simulink model "PID_Validation_Luca"  (R2024b)
settings: Solver=ode45  StartTime=0.0  StopTime=4  RelTol=1e-3
values from neighbouring files (symbols this model uses):
  Beq = mot.B+(mld.Bh)/((gbox.N)^2)    [LQR_code.m]
  Jb = 1.4e-3    (= 0.0014)    [Elastic_parameters_estimation.m]
  Kd = Kp * TD    [PID.m]
  Ki = Kp / TI    [PID.m]
  Kp = 1/(magP * magC)    [PID.m]
  Kw = 1/T_w    (= 7.14285714286)    [PID_Luca.m]
  N = linsolve(SYS,f)    [LQR_code.m]
  Req = sens.curr.Rs+mot.R    [LQR_code.m]
  tl = 1/(10*wgc)    [PID_Luca.m]
undefined symbols (not defined in the file or in its folder): Bb, daq, deg2V, drv, Jeq_hat, k, k_drv, Ke, Kt, mot, rads2rpm, sens, T_drv, tau_sf, V2deg
settings Model: Creator=Banaan  LastModifiedBy=lucag

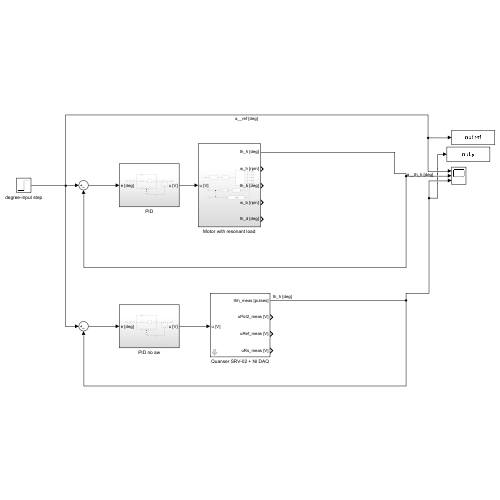
[thumbnail: Simulink's stored preview of the top-level diagram]
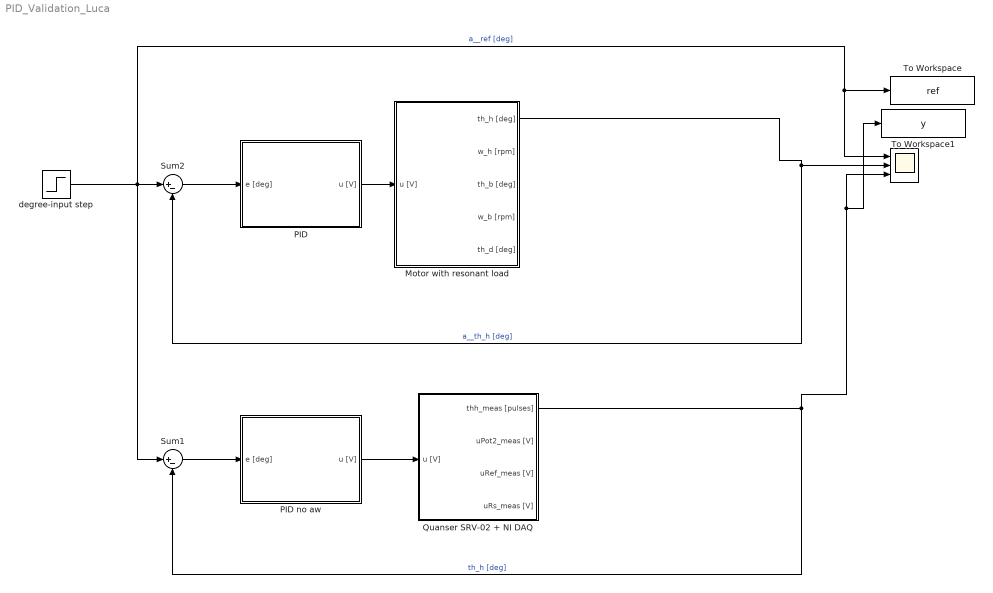
== system PID_Validation_Luca ==
  " " : Scope  NumInputPorts=3
  Motor with resonant load : Subsystem
  PID : Subsystem
  PID no aw : Subsystem
  Quanser SRV-02 + NI DAQ : Subsystem  mask(Quanser SRV-02 (with resonant load) + NI DAQ){Ts=0.001, fricType=Coulomb + viscous, lockShaft=off, beamInitPos=10}
      mask prompts: Ts "NI DAQ Sample Time:"; fricType "Friction model"; lockShaft "Lock motor shaft"; beamInitPos "Beam initial position [deg]:"
      mask help: Quanser SRV-02 (with resonant load) + NI DAQ model.
      mask init:
      | %%
      | % Riccardo Antonello (riccardo.antonello@unipd.it)
      | %
      | % April 28, 2020
      | %
      | % Dept. of Information Engineering, University of Padova
      | %
      | 
      | %%  Conversion gains
      | deg2rad = pi/180;                   %   [deg]   -> [rad]
      | rad2deg = 180/pi;                   %   [rad]   -> [deg]
      | 
      | 
      | %%  Sensors data
      | 
      | %   shunt resistor
      | sens.curr.Rs = 0.5;   
      | 
      | %   Hewlett-Packard HEDS-5540#A06 optical encoder
      | sens.enc.ppr = 500*4;                                                   %   pulses per rotation
      | sens.enc.pulse2deg = 360/sens.enc.ppr;                                  %   [pulses] -> [deg]
      | sens.enc.pulse2rad = 2*pi/sens.enc.ppr;                                 %   [pulses] -> [rad]
      | sens.enc.deg2pulse = sens.enc.ppr/360;                                  %   [deg] -> [pulses]
      | sens.enc.rad2pulse = sens.enc.ppr/2/pi;                                 %   [rad] -> [pulses]
      | 
      | %   potentiometer 2 (Spectrol 357-0-0-103) - installed on hub
      | sens.pot2.range.R      = 10e3;                                          %   ohmic value range 
      | sens.pot2.range.V      = 5;                                             %   voltage range
      | sens.pot2.range.th_deg = 340;                                           %   angle range [deg]
      | sens.pot2.range.th     = sens.pot2.range.th_deg * deg2rad;              %   angle range [rad]                           
      | sens.pot2.deg2V        = sens.pot2.range.V / sens.pot2.range.th_deg;    %   sensitivity [V/deg]
      | sens.pot2.rad2V        = sens.pot2.range.V / sens.pot2.range.th;        %   sensitivity [V/rad]
      | sens.pot2.V2deg        = 1/sens.pot2.deg2V;                             %   conversion gain [V] -> [deg]
      | sens.pot2.V2rad        = 1/sens.pot2.rad2V;                             %   conversion gain [V] -> [rad]
      | sens.pot2.noise.var    = 3.5e-7;                                        %   out noise variance [V^2]
      | 
      | 
      | %%  Data acquisition board (daq) data
      | 
      | %   NI PCI-6221 DAC data
      | daq.dac.bits = 16;                                  %   resolution (bits)
      | daq.dac.fs   = 10;                                  %   full scale 
      | daq.dac.q    = 2*daq.dac.fs/(2^daq.dac.bits-1);     %	quantization
      | 
      | %   NI PCI-6221 ADC data
      | daq.adc.bits = 16;                                  %   resolution (bits)
      | daq.adc.fs   = 10;                                  %   full scale (as set in SLDRT Analog Input block)
      | daq.adc.q    = 2*daq.adc.fs/(2^daq.adc.bits-1);     %   quantization   
      | 
      | 
      | %%  Set beam initial position
      | % SRV02Handle = find_system(gcb, ...
      | %     'LookUnderMasks', 'on', ...
      | %     'FindAll', 'on', ...
      | %     'FollowLinks', 'on', ...
      | %     'SearchDepth', '1', ...
      | %     'BlockType', 'ModelReference', ...
      | %     'Name', 'Quanser SRV-02');
      | %
      | % %get_param(SRV02Handle, 'InstanceParameters')
      | % InstanceParams = get_param(SRV02Handle, 'InstanceParameters');
      | % for k = 1:length(InstanceParams)
      | %     if strcmp(InstanceParams(k).Name, 'thb0')
      | %         if lockShaft
      | %             InstanceParams(k).Value = sprintf('%f', beamInitPos);
      | %         else
      | %             InstanceParams(k).Value = sprintf('%f', 0);    
      | %         end
      | %         set_param(SRV02Handle, 'InstanceParameters', InstanceParams);
      | %         break;
      | %     end
      | % end
      | 
      | if lockShaft
      |     thb0 = beamInitPos;
      | else
      |     thb0 = 0;    
      | end
      | 
      | 
      | %%  Mask initialization
      | if lockShaft
      |     
      |     %   find Inport handle
      |     InPortHandle = find_system(gcb, ...
      |         'LookUnderMasks', 'on', ...
      |         'FindAll', 'on', ...
      |         'FollowLinks', 'on', ...
      |         'SearchDepth', '1', ...
      |         'BlockType', 'Inport', ...
      |         'Name', 'u [V]');
      |     
      |     if ~isempty(InPortHandle)
      |     
      |         %   find DAC handle
      |         DACHandle = find_system(gcb, ...
      |             'LookUnderMasks', 'on', ...
      |             'FindAll', 'on', ...
      |             'FollowLinks', 'on', ...
      |             'SearchDepth', '1', ...
      |             'BlockType', 'SubSystem', ...
      |             'Name', 'DAC');  
      | 
      |         %   remove Inport output connection   
      |         InportConn = get_param(InPortHandle, 'PortConnectivity');
      |         delete_line(gcb, InportConn.Position);
      | 
      |         %   remove Inport block
      |         delete_block(InPortHandle);
      | 
      |         %   add Constant block
      |         ConstantHandle = add_block( ...
      |             'simulink/Sources/Constant', [gcb, '/u [V]'], ...
      |             'Position', [20   -37    50   -23], ...
      |             'Value', '0');
      | 
      |         %   connect Constant to DAC block
      |         DACPortHandles = get_param(DACHandle, 'PortHandles');
      |         ConstantPortHandles = get_param(ConstantHandle, 'PortHandles');
      |         add_line(gcb, ConstantPortHandles.Outport(1), DACPortHandles.Inport(1));
      |     
      |     end
      |     
      | else
      |     
      |     %   find Constant handle
      |     ConstantHandle = find_system(gcb, ...
      |         'LookUnderMasks', 'on', ...
      |         'FindAll', 'on', ...
      |         'FollowLinks', 'on', ...
      |         'SearchDepth', '1', ...
      |         'BlockType', 'Constant', ...
      |         'Name', 'u [V]');
      |     
      |     if ~isempty(ConstantHandle)
      |     
      |         %   find DAC handle
      |         DACHandle = find_system(gcb, ...
      |             'LookUnderMasks', 'on', ...
      |             'FindAll', 'on', ...
      |             'FollowLinks', 'on', ...
      |             'SearchDepth', '1', ...
      |             'BlockType', 'SubSystem', ...
      |             'Name', 'DAC');  
      |  
      |         %   remove Constant output connection   
      |         ConstantConn = get_param(ConstantHandle, 'PortConnectivity');
      |         delete_line(gcb, ConstantConn.Position);
      | 
      |         %   remove Inport block
      |         delete_block(ConstantHandle);   
      | 
      |         %   add Inport block
      |         InportHandle = add_block( ...
      |             'simulink/Sources/In1', [gcb, '/u [V]'], ...
      |             'Position', [20   -37    50   -23], ...
      |             'Port', '1');
      | 
      |         %   connect Constant to DAC block
      |         DACPortHandles = get_param(DACHandle, 'PortHandles');
      |         InportPortHandles = get_param(InportHandle, 'PortHandles');
      |         add_line(gcb, InportPortHandles.Outport(1), DACPortHandles.Inport(1));
      |     
      |      end
      |     
      | end
      mask Help:
      | Riccardo Antonello (antonello@dei.unipd.it)
      | 
      | April 28, 2020
      | 
      | Dept. of Information Engineering, University of Padova
      mask TypeOptions fricType: Coulomb + viscous | Karnopp
      mask Callback lockShaft:
      | %   get status of check box
      | lockShaft = get_param(gcb, 'lockShaft');
      | 
      | %   get current value of MaskVisibilities property
      | maskVisibilities = get_param(gcb, 'MaskVisibilities');
      | 
      | %   set visibility of the dialog box element
      | if strcmp(lockShaft, 'on')
      |     maskVisibilities{4} = 'on';
      | else
      |     maskVisibilities{4} = 'off';
      | end
      | 
      | % Set the 'MaskVisibilities' property for each parameter in mask
      | set_param( gcb, 'MaskVisibilities', maskVisibilities);
  Sum1 : Sum  Inputs=|+-
  Sum2 : Sum  Inputs=|+-
  To Workspace : ToWorkspace  VariableName=ref  SaveFormat=Structure With Time  SampleTime=-1
  To Workspace1 : ToWorkspace  VariableName=y  SaveFormat=Structure With Time  SampleTime=-1
  degree-input step : Step  Time=0  After=100  SampleTime=0
  wires:
  degree-input step/1 -> Sum1/1, Sum2/1, " "/1, To Workspace/1  "a__ref [deg]"
  Sum2/1 -> PID/1(e [deg])
  PID/1(u [V]) -> Motor with resonant load/1(u [V])
  Motor with resonant load/1(th_h [deg]) -> Sum2/2, " "/2  "a__th_h [deg]"
  PID no aw/1(u [V]) -> Quanser SRV-02 + NI DAQ/1(u [V])
  Sum1/1 -> PID no aw/1(e [deg])
  Quanser SRV-02 + NI DAQ/1(thh_meas [pulses]) -> To Workspace1/1, " "/3, Sum1/2  "th_h [deg]"

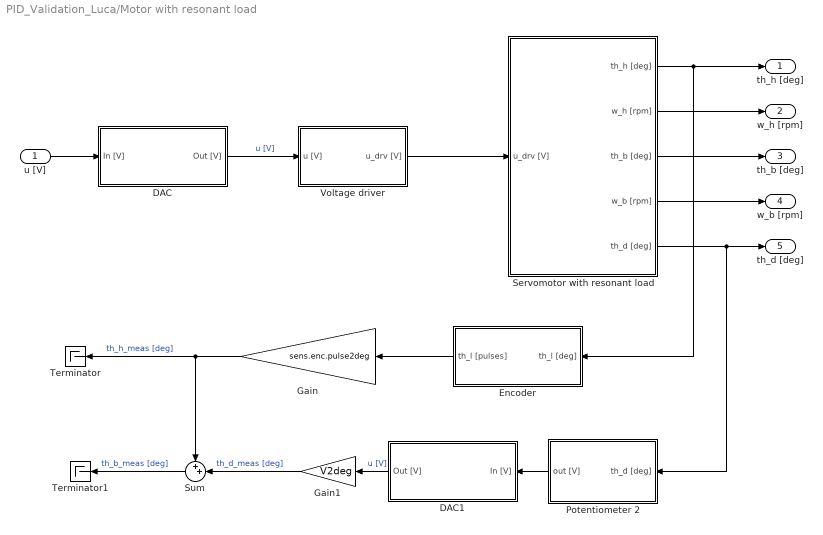
== system PID_Validation_Luca/Motor with resonant load ==
  u [V] : Inport
  DAC : Subsystem
  DAC1 : Subsystem
  Encoder : Subsystem
  Gain : Gain  Gain=sens.enc.pulse2deg
  Gain1 : Gain  Gain=V2deg
  Potentiometer 2 : Subsystem
  Servomotor with resonant load : Subsystem
  Sum : Sum  Inputs=++|
  Terminator : Terminator
  Terminator1 : Terminator
  Voltage driver : Subsystem
  th_h [deg] : Outport
  w_h [rpm] : Outport  Port=2
  th_b [deg] : Outport  Port=3
  w_b [rpm] : Outport  Port=4
  th_d [deg] : Outport  Port=5
  wires:
  Encoder/1(th_l [pulses]) -> Gain/1
  u [V]/1 -> DAC/1(In [V])
  DAC/1(Out [V]) -> Voltage driver/1(u [V])  "u [V]"
  Voltage driver/1(u_drv [V]) -> Servomotor with resonant load/1(u_drv [V])
  Servomotor with resonant load/1(th_h [deg]) -> Encoder/1(th_l [deg]), th_h [deg]/1
  Servomotor with resonant load/2(w_h [rpm]) -> w_h [rpm]/1
  Servomotor with resonant load/3(th_b [deg]) -> th_b [deg]/1
  Servomotor with resonant load/4(w_b [rpm]) -> w_b [rpm]/1
  Servomotor with resonant load/5(th_d [deg]) -> Potentiometer 2/1(th_d [deg]), th_d [deg]/1
  Gain/1 -> Terminator/1, Sum/1  "th_h_meas [deg]"
  Potentiometer 2/1(out [V]) -> DAC1/1(In [V])
  DAC1/1(Out [V]) -> Gain1/1  "u [V]"
  Gain1/1 -> Sum/2  "th_d_meas [deg]"
  Sum/1 -> Terminator1/1  "th_b_meas [deg]"

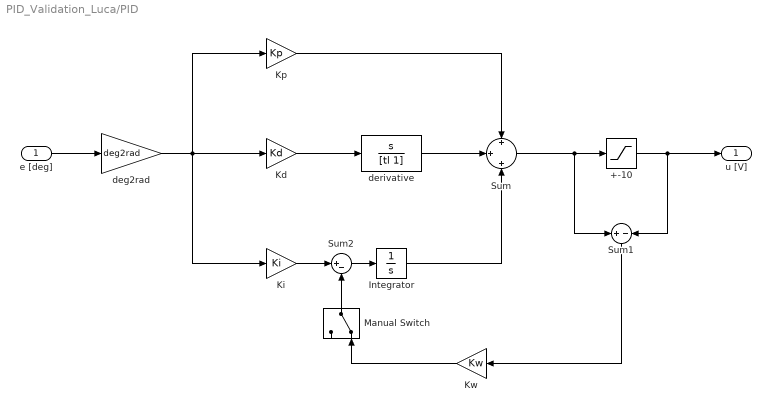
== system PID_Validation_Luca/PID ==
  e [deg] : Inport
  +-10 : Saturate  UpperLimit=10  LowerLimit=-10
  Integrator : Integrator
  Kd : Gain  Gain=Kd
  Ki : Gain  Gain=Ki
  Kp : Gain  Gain=Kp
  Kw : Gain  Gain=Kw
  Manual Switch : ManualSwitch  CurrentSetting=0
  Sum : Sum  Inputs=+|+|+
  Sum1 : Sum  Inputs=+|-
  Sum2 : Sum  Inputs=|+-
  deg2rad : Gain  Gain=deg2rad
  derivative : TransferFcn  Numerator=[1 0]  Denominator=[tl 1]
  u [V] : Outport
  wires:
  +-10/1 -> u [V]/1, Sum1/2
  derivative/1 -> Sum/2
  deg2rad/1 -> Kp/1, Ki/1, Kd/1
  Kp/1 -> Sum/1
  Ki/1 -> Sum2/1
  Sum/1 -> Sum1/1, +-10/1
  Manual Switch/1 -> Sum2/2
  Sum1/1 -> Kw/1
  Kd/1 -> derivative/1
  e [deg]/1 -> deg2rad/1
  Sum2/1 -> Integrator/1
  Integrator/1 -> Sum/3
  Kw/1 -> Manual Switch/2

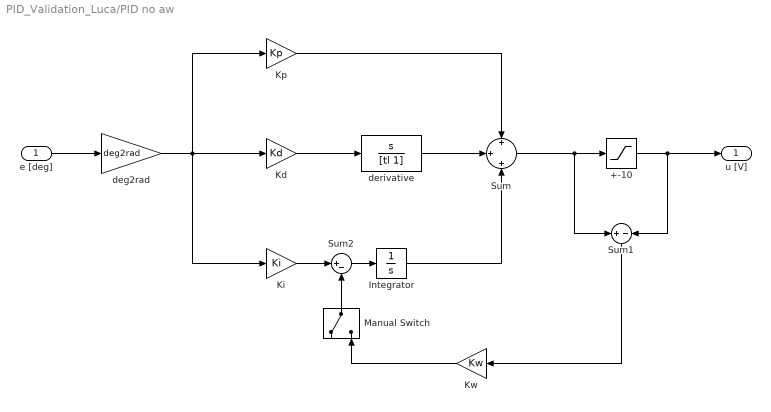
== system PID_Validation_Luca/PID no aw ==
  e [deg] : Inport
  +-10 : Saturate  UpperLimit=10  LowerLimit=-10
  Integrator : Integrator
  Kd : Gain  Gain=Kd
  Ki : Gain  Gain=Ki
  Kp : Gain  Gain=Kp
  Kw : Gain  Gain=Kw
  Manual Switch : ManualSwitch
  Sum : Sum  Inputs=+|+|+
  Sum1 : Sum  Inputs=+|-
  Sum2 : Sum  Inputs=|+-
  deg2rad : Gain  Gain=deg2rad
  derivative : TransferFcn  Numerator=[1 0]  Denominator=[tl 1]
  u [V] : Outport
  wires:
  Kw/1 -> Manual Switch/2
  Integrator/1 -> Sum/3
  Sum2/1 -> Integrator/1
  e [deg]/1 -> deg2rad/1
  Kd/1 -> derivative/1
  Sum1/1 -> Kw/1
  Manual Switch/1 -> Sum2/2
  Sum/1 -> +-10/1, Sum1/1
  Ki/1 -> Sum2/1
  Kp/1 -> Sum/1
  deg2rad/1 -> Kd/1, Ki/1, Kp/1
  derivative/1 -> Sum/2
  +-10/1 -> Sum1/2, u [V]/1

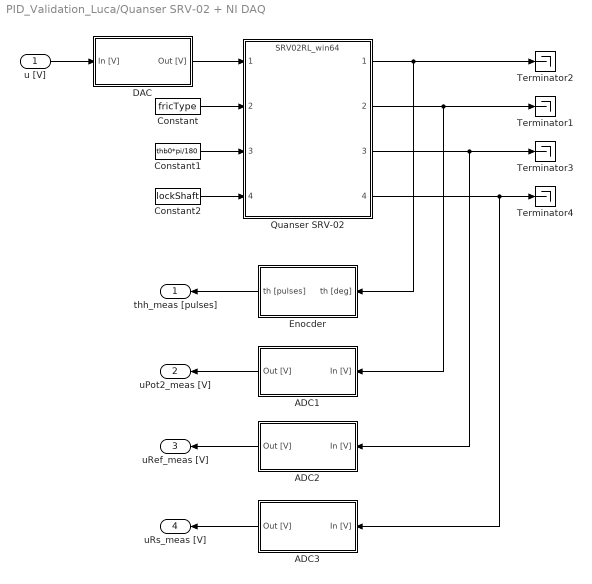
== system PID_Validation_Luca/Quanser SRV-02 + NI DAQ ==
  u [V] : Inport
  ADC1 : Subsystem
  ADC2 : Subsystem
  ADC3 : Subsystem
  Constant : Constant  Value=fricType
  Constant1 : Constant  Value=thb0*pi/180  SampleTime=Inf
  Constant2 : Constant  Value=lockShaft  SampleTime=Inf
  DAC : Subsystem
  Enocder : Subsystem
  Quanser SRV-02 : ModelReference  ModelNameDialog=SRV02RL_win64.slxp  ModelReferenceVersion=1.76  CopyOfModelProtected=on
  Terminator{1..4} (4 alike) : Terminator
  thh_meas [pulses] : Outport
  uPot2_meas [V] : Outport  Port=2
  uRef_meas [V] : Outport  Port=3
  uRs_meas [V] : Outport  Port=4
  wires:
  Enocder/1(th [pulses]) -> thh_meas [pulses]/1
  ADC3/1(Out [V]) -> uRs_meas [V]/1
  DAC/1(Out [V]) -> Quanser SRV-02/1
  Quanser SRV-02/2 -> ADC1/1(In [V]), Terminator1/1
  Quanser SRV-02/1 -> Terminator2/1, Enocder/1(th [deg])
  Constant/1 -> Quanser SRV-02/2
  Quanser SRV-02/3 -> ADC2/1(In [V]), Terminator3/1
  ADC1/1(Out [V]) -> uPot2_meas [V]/1
  Constant1/1 -> Quanser SRV-02/3
  Constant2/1 -> Quanser SRV-02/4
  Quanser SRV-02/4 -> ADC3/1(In [V]), Terminator4/1
  ADC2/1(Out [V]) -> uRef_meas [V]/1
  u [V]/1 -> DAC/1(In [V])

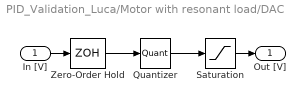
== system PID_Validation_Luca/Motor with resonant load/DAC ==
  In [V] : Inport
  Quantizer : Quantizer  QuantizationInterval=daq.dac.q
  Saturation : Saturate  UpperLimit=daq.dac.fs  LowerLimit=-daq.dac.fs
  Zero-Order Hold : ZeroOrderHold  SampleTime=1e-3
  Out [V] : Outport
  wires:
  Saturation/1 -> Out [V]/1
  Zero-Order Hold/1 -> Quantizer/1
  Quantizer/1 -> Saturation/1
  In [V]/1 -> Zero-Order Hold/1

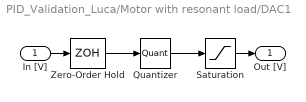
== system PID_Validation_Luca/Motor with resonant load/DAC1 ==
  In [V] : Inport
  Quantizer : Quantizer  QuantizationInterval=daq.dac.q
  Saturation : Saturate  UpperLimit=daq.dac.fs  LowerLimit=-daq.dac.fs
  Zero-Order Hold : ZeroOrderHold  SampleTime=1e-3
  Out [V] : Outport
  wires:
  In [V]/1 -> Zero-Order Hold/1
  Quantizer/1 -> Saturation/1
  Zero-Order Hold/1 -> Quantizer/1
  Saturation/1 -> Out [V]/1

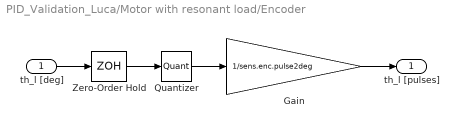
== system PID_Validation_Luca/Motor with resonant load/Encoder ==
  th_l [deg] : Inport
  Gain : Gain  Gain=1/sens.enc.pulse2deg
  Quantizer : Quantizer  QuantizationInterval=sens.enc.pulse2deg
  Zero-Order Hold : ZeroOrderHold  SampleTime=1e-3
  th_l [pulses] : Outport
  wires:
  th_l [deg]/1 -> Zero-Order Hold/1
  Quantizer/1 -> Gain/1
  Zero-Order Hold/1 -> Quantizer/1
  Gain/1 -> th_l [pulses]/1

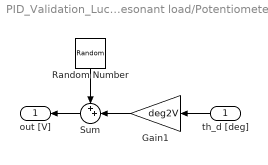
== system PID_Validation_Luca/Motor with resonant load/Potentiometer 2 ==
  th_d [deg] : Inport
  Gain1 : Gain  Gain=deg2V
  Random Number : RandomNumber  Variance=sens.pot2.noise.var  SampleTime=1e-3
  Sum : Sum  Inputs=++|
  out [V] : Outport
  wires:
  Gain1/1 -> Sum/2
  th_d [deg]/1 -> Gain1/1
  Random Number/1 -> Sum/1
  Sum/1 -> out [V]/1

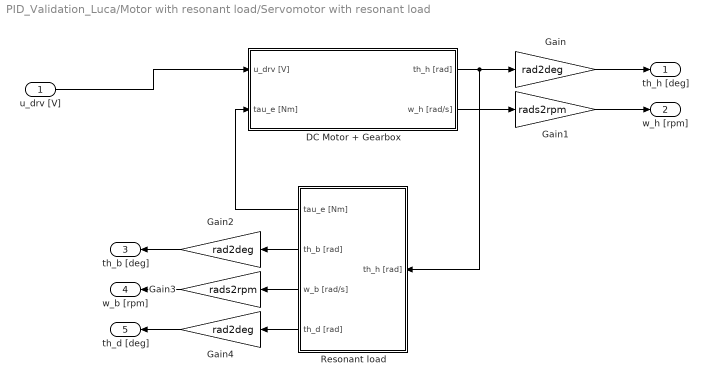
== system PID_Validation_Luca/Motor with resonant load/Servomotor with resonant load ==
  u_drv [V] : Inport
  DC Motor + Gearbox : Subsystem
  Gain : Gain  Gain=rad2deg
  Gain1 : Gain  Gain=rads2rpm
  Gain2 : Gain  Gain=rad2deg
  Gain3 : Gain  Gain=rads2rpm
  Gain4 : Gain  Gain=rad2deg
  Resonant load : Subsystem
  th_h [deg] : Outport
  w_h [rpm] : Outport  Port=2
  th_b [deg] : Outport  Port=3
  w_b [rpm] : Outport  Port=4
  th_d [deg] : Outport  Port=5
  wires:
  Resonant load/1(tau_e [Nm]) -> DC Motor + Gearbox/2(tau_e [Nm])
  Gain4/1 -> th_d [deg]/1
  Gain2/1 -> th_b [deg]/1
  Resonant load/2(th_b [rad]) -> Gain2/1
  DC Motor + Gearbox/2(w_h [rad/s]) -> Gain1/1
  DC Motor + Gearbox/1(th_h [rad]) -> Gain/1, Resonant load/1(th_h [rad])
  Resonant load/3(w_b [rad/s]) -> Gain3/1
  Gain1/1 -> w_h [rpm]/1
  Resonant load/4(th_d [rad]) -> Gain4/1
  Gain/1 -> th_h [deg]/1
  Gain3/1 -> w_b [rpm]/1
  u_drv [V]/1 -> DC Motor + Gearbox/1(u_drv [V])

== system PID_Validation_Luca/Motor with resonant load/Voltage driver ==
  u [V] : Inport
  Driver dynamics : TransferFcn  Numerator=[k_drv]  Denominator=[T_drv 1]
  Driver saturation : Saturate  UpperLimit=drv.outmax  LowerLimit=-drv.outmax
  u_drv [V] : Outport
  wires:
  Driver dynamics/1 -> Driver saturation/1
  Driver saturation/1 -> u_drv [V]/1
  u [V]/1 -> Driver dynamics/1

== system PID_Validation_Luca/Quanser SRV-02 + NI DAQ/ADC1 ==
  In [V] : Inport
  ADC quantization : Quantizer  QuantizationInterval=daq.adc.q
  ADC sampling : ZeroOrderHold  SampleTime=Ts
  ADC saturation : Saturate  UpperLimit=daq.adc.fs  LowerLimit=-daq.adc.fs
  Out [V] : Outport
  wires:
  ADC saturation/1 -> Out [V]/1
  ADC sampling/1 -> ADC quantization/1
  In [V]/1 -> ADC sampling/1
  ADC quantization/1 -> ADC saturation/1

== system PID_Validation_Luca/Quanser SRV-02 + NI DAQ/ADC2 ==
  In [V] : Inport
  ADC quantization : Quantizer  QuantizationInterval=daq.adc.q
  ADC sampling : ZeroOrderHold  SampleTime=Ts
  ADC saturation : Saturate  UpperLimit=daq.adc.fs  LowerLimit=-daq.adc.fs
  Out [V] : Outport
  wires:
  ADC quantization/1 -> ADC saturation/1
  In [V]/1 -> ADC sampling/1
  ADC sampling/1 -> ADC quantization/1
  ADC saturation/1 -> Out [V]/1

== system PID_Validation_Luca/Quanser SRV-02 + NI DAQ/ADC3 ==
  In [V] : Inport
  Quantizer : Quantizer  QuantizationInterval=daq.adc.q
  Saturation : Saturate  UpperLimit=daq.adc.fs  LowerLimit=-daq.adc.fs
  Zero-Order Hold : ZeroOrderHold  SampleTime=Ts
  Out [V] : Outport
  wires:
  Saturation/1 -> Out [V]/1
  In [V]/1 -> Zero-Order Hold/1
  Quantizer/1 -> Saturation/1
  Zero-Order Hold/1 -> Quantizer/1

== system PID_Validation_Luca/Quanser SRV-02 + NI DAQ/DAC ==
  In [V] : Inport
  Quantizer : Quantizer  QuantizationInterval=daq.dac.q
  Saturation : Saturate  UpperLimit=daq.dac.fs  LowerLimit=-daq.dac.fs
  Zero-Order Hold : ZeroOrderHold  SampleTime=Ts
  Out [V] : Outport
  wires:
  Quantizer/1 -> Saturation/1
  In [V]/1 -> Zero-Order Hold/1
  Zero-Order Hold/1 -> Quantizer/1
  Saturation/1 -> Out [V]/1

== system PID_Validation_Luca/Quanser SRV-02 + NI DAQ/Enocder ==
  th [deg] : Inport
  Quantizer : Quantizer  QuantizationInterval=sens.enc.pulse2deg
  Zero-Order Hold : ZeroOrderHold  SampleTime=Ts
  deg2pulse : Gain  Gain=sens.enc.deg2pulse
  th [pulses] : Outport
  wires:
  Quantizer/1 -> deg2pulse/1
  th [deg]/1 -> Zero-Order Hold/1
  Zero-Order Hold/1 -> Quantizer/1
  deg2pulse/1 -> th [pulses]/1

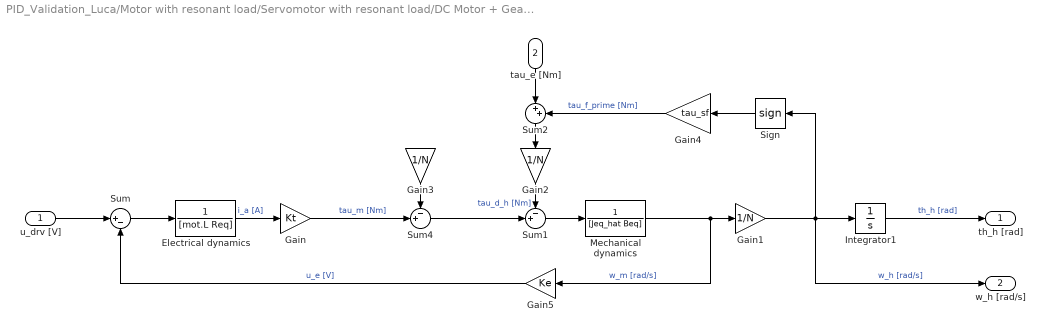
== system PID_Validation_Luca/Motor with resonant load/Servomotor with resonant load/DC Motor + Gearbox ==
  u_drv [V] : Inport
  tau_e [Nm] : Inport  Port=2
  Electrical dynamics : TransferFcn  Denominator=[mot.L Req]
  Gain : Gain  Gain=Kt
  Gain1 : Gain  Gain=1/N
  Gain2 : Gain  Gain=1/N
  Gain3 : Gain  Gain=1/N
  Gain4 : Gain  Gain=tau_sf
  Gain5 : Gain  Gain=Ke
  Integrator1 : Integrator
  Mechanical dynamics : TransferFcn  Denominator=[Jeq_hat Beq]
  Sign : Signum  ZeroCross=off
  Sum : Sum  Inputs=|+-
  Sum1 : Sum  Inputs=-+|
  Sum2 : Sum  Inputs=|++
  Sum4 : Sum  Inputs=-+|
  th_h [rad] : Outport
  w_h [rad/s] : Outport  Port=2
  wires:
  Integrator1/1 -> th_h [rad]/1  "th_h [rad]"
  Gain5/1 -> Sum/2  "u_e [V]"
  Gain1/1 -> Sign/1, w_h [rad/s]/1, Integrator1/1  "w_h [rad/s]"
  Electrical dynamics/1 -> Gain/1  "i_a [A]"
  Sign/1 -> Gain4/1
  Sum/1 -> Electrical dynamics/1
  Sum1/1 -> Mechanical dynamics/1
  Gain/1 -> Sum4/2  "tau_m [Nm]"
  Mechanical dynamics/1 -> Gain5/1, Gain1/1  "w_m [rad/s]"
  u_drv [V]/1 -> Sum/1
  Gain4/1 -> Sum2/2  "tau_f_prime [Nm]"
  Sum2/1 -> Gain2/1
  tau_e [Nm]/1 -> Sum2/1
  Gain2/1 -> Sum1/1  "tau_d_h [Nm]"
  Sum4/1 -> Sum1/2
  Gain3/1 -> Sum4/1

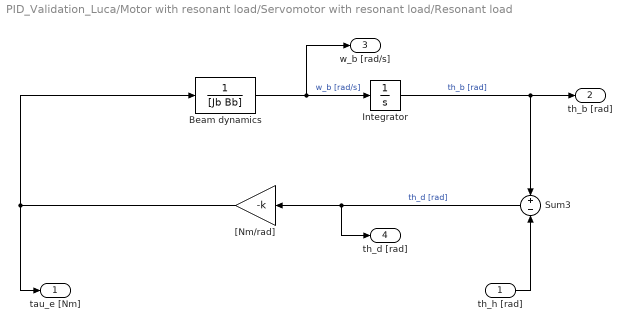
== system PID_Validation_Luca/Motor with resonant load/Servomotor with resonant load/Resonant load ==
  th_h [rad] : Inport
  Beam dynamics : TransferFcn  Denominator=[Jb Bb]
  Integrator : Integrator
  Sum3 : Sum  Inputs=+|-
  "[Nm/rad]" : Gain  Gain=-k
  tau_e [Nm] : Outport
  th_b [rad] : Outport  Port=2
  w_b [rad/s] : Outport  Port=3
  th_d [rad] : Outport  Port=4
  wires:
  Integrator/1 -> th_b [rad]/1, Sum3/1  "th_b [rad]"
  "[Nm/rad]"/1 -> tau_e [Nm]/1, Beam dynamics/1
  Sum3/1 -> th_d [rad]/1, "[Nm/rad]"/1  "th_d [rad]"
  Beam dynamics/1 -> w_b [rad/s]/1, Integrator/1  "w_b [rad/s]"
  th_h [rad]/1 -> Sum3/2
